simulink model "ASLIPrun2"  (R2015a)
settings: Solver=ode45  StartTime=0.0  StopTime=simtime  MaxStep=1e-3  RelTol=1e-4  AbsTol=1e-6
values from neighbouring files (symbols this model uses):
  a0 = 68*pi/180    (= 1.18682389136)    [smm_params.m]
  dt0 = -0.3325    [SLIPquad_params.m]
  dx0 = 0.4138    [SLIPquad_params.m]    (also in SLIPrun_params.m = 3; SLIPwalk_params.m = 2.5; smm_params.m = 5)
  dy0 = 0.1683    [SLIPquad_params.m]    (also in SLIPrun_params.m = -1; SLIPwalk_params.m = 0; smm_params.m = 0)
  g = 1    [SLIPquad_params.m]    (also in SLIPrun_params.m = 9.81; SLIPwalk_params.m = 9.81; smm_params.m = 9.81)
  J = 0.6    [SLIPquad_params.m]
  k = 20    [SLIPquad_params.m]    (also in SLIPrun_params.m = 23000; SLIPwalk_params.m = 10000; smm_params.m = 20000)
  L = sqrt( (u(3)-u(1))^2 + (u(4)-u(2))^2 )    [AnimSMR.m]    (also in SLIPquad_params.m = 0.5)
  l0 = 1    [SLIPquad_params.m]    (also in SLIPrun_params.m; SLIPwalk_params.m; smm_params.m)
  m = 1    [SLIPquad_params.m]    (also in SLIPrun_params.m = 70; SLIPwalk_params.m = 70; smm_params.m = 80)
  t0 = 0.056    [SLIPquad_params.m]
  x0 = []    [AnimQUAD.m]    (also in AnimQUAD2.m; AnimSMR.m; SLIPquad_params.m = 0; SLIPrun_params.m = -l*sin(theta_th))
  y0 = 1.0237    [SLIPquad_params.m]    (also in SLIPrun_params.m = sqrt(l^2 - x0^2); SLIPwalk_params.m = sqrt(l0^2 - x0^2); smm_params.m = 1)
libraries: simulink_extras x1
settings Model: Creator=hgeyer  LastModifiedBy=Joe
settings DataIOCC: SignalLoggingSaveFormat=ModelDataLogs
settings OptimizationCC: ExpressionDepthLimit=2147483647
settings DebuggingCC: UnderspecifiedInitializationDetection=Classic  MergeDetectMultiDrivingBlocksExec=none  SolverPrmCheckMsg=warning  FcnCallInpInsideContextMsg=EnableAllAsWarning  StateNameClashWarn=warning

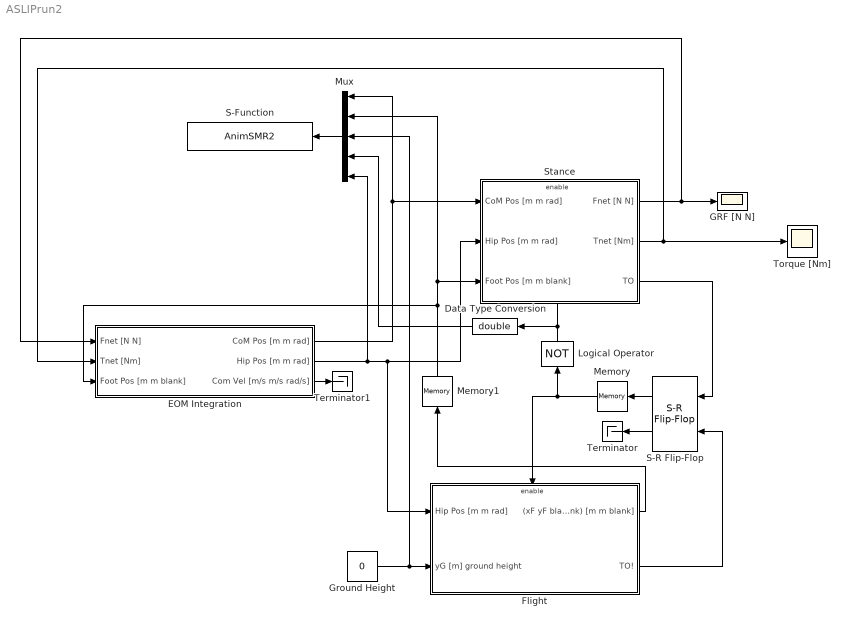
== system ASLIPrun2 ==
  Data Type Conversion : DataTypeConversion  OutDataTypeStr=double
  EOM Integration : Subsystem
  Flight : Subsystem
  GRF [N N] : Scope
      settings: YMin=-10  YMax=10
  Ground Height : Constant  Value=0
  Logical Operator : Logic  Operator=NOT  AllPortsSameDT=off  OutDataTypeStr=boolean
  Memory : Memory  X0=1
  Memory1 : Memory  X0=[0 0 0]
  Mux : Mux  Inputs=5
  S-Function : S-Function  FunctionName=AnimSMR2  Parameters=0.002
  S-R Flip-Flop : simulink_extras/Flip Flops/S-R Flip-Flop  initial_condition=1
  Stance : Subsystem
  Terminator : Terminator
  Terminator1 : Terminator
  Torque [Nm] : Scope
      settings: YMin=-10  YMax=10  SaveName=ScopeData3
  wires:
  EOM Integration/1(CoM Pos [m m rad]) -> Stance/1("CoM Pos [m m rad] "), Mux/1
  Stance/3(TO) -> S-R Flip-Flop/1
  S-R Flip-Flop/1 -> Memory/1
  Logical Operator/1 -> Data Type Conversion/1, Stance/Enable
  Memory/1 -> Logical Operator/1, Flight/Enable
  Flight/2(TO!) -> S-R Flip-Flop/2
  Stance/1(Fnet [N N]) -> EOM Integration/1(Fnet [N N]), GRF [N N]/1
  Flight/1((xF yF blank) [m m blank]) -> Memory1/1
  Memory1/1 -> EOM Integration/3(Foot Pos [m m blank]), Mux/2, Stance/3(Foot Pos [m m blank])
  Mux/1 -> S-Function/1
  S-R Flip-Flop/2 -> Terminator/1
  Ground Height/1 -> Mux/3, Flight/2(yG [m] ground height)
  EOM Integration/3(Com Vel [m/s m/s rad/s]) -> Terminator1/1
  Data Type Conversion/1 -> Mux/4
  EOM Integration/2(Hip Pos [m m rad]) -> Mux/5, Stance/2(Hip Pos [m m rad]), Flight/1(Hip Pos [m m rad])
  Stance/2(Tnet [Nm]) -> Torque [Nm]/1, EOM Integration/2(Tnet [Nm])

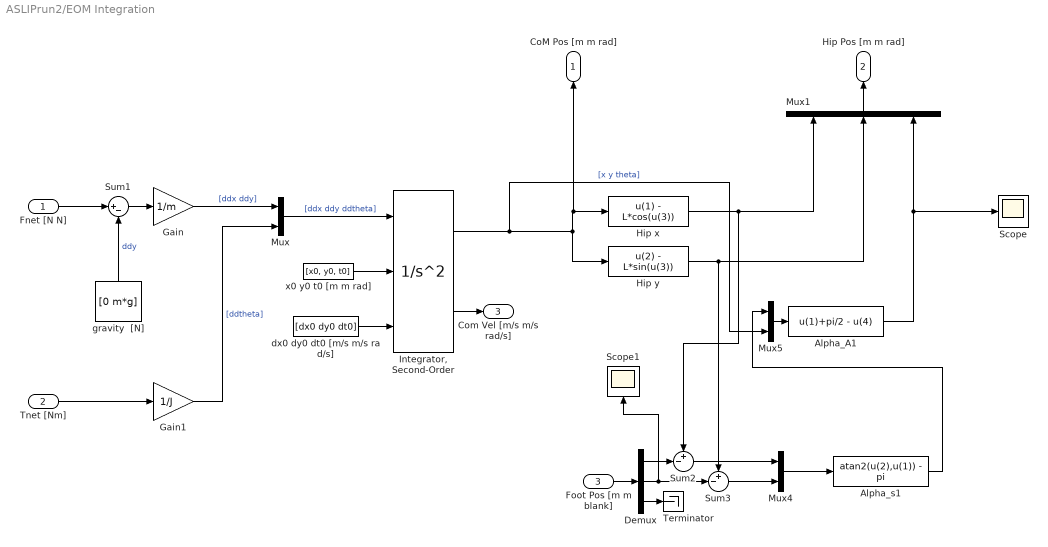
== system ASLIPrun2/EOM Integration ==
  Fnet [N N] : Inport
  Tnet [Nm] : Inport  Port=2
  Foot Pos [m m blank] : Inport  Port=3
  Alpha_A1 : Fcn  Expr=u(1)+pi/2 - u(4)
  Alpha_s1 : Fcn  Expr=atan2(u(2),u(1)) - pi
  Demux : Demux  Outputs=3
  Gain : Gain  Gain=1/m
  Gain1 : Gain  Gain=1/J
  Hip x : Fcn  Expr=u(1) - L*cos(u(3))
  Hip y : Fcn  Expr=u(2) - L*sin(u(3))
  "Integrator, Second-Order" : SecondOrderIntegrator  ICSourceX=external  ICSourceDXDT=external
  Mux : Mux  Inputs=2
  Mux1 : Mux  Inputs=3
  Mux4 : Mux  Inputs=2
  Mux5 : Mux  Inputs=2
  Scope : Scope
      settings: SaveName=ScopeData2
  Scope1 : Scope
  Sum1 : Sum  Inputs=|+-
  Sum2 : Sum  Inputs=+-|
  Sum3 : Sum  Inputs=+-|
  Terminator : Terminator
  dx0 dy0 dt0 [m/s m/s ra d/s] : Constant  Value=[dx0 dy0 dt0]
  gravity  [N] : Constant  Value=[0 m*g]
  x0 y0 t0 [m m rad] : Constant  Value=[x0, y0, t0]
  CoM Pos [m m rad] : Outport
  Hip Pos [m m rad] : Outport  Port=2
  Com Vel [m/s m/s rad/s] : Outport  Port=3
  wires:
  Sum1/1 -> Gain/1
  gravity  [N]/1 -> Sum1/2  "ddy"
  x0 y0 t0 [m m rad]/1 -> "Integrator, Second-Order"/2
  Gain/1 -> Mux/1  "[ddx ddy]"
  Fnet [N N]/1 -> Sum1/1
  dx0 dy0 dt0 [m/s m/s ra d/s]/1 -> "Integrator, Second-Order"/3
  Mux/1 -> "Integrator, Second-Order"/1  "[ddx ddy ddtheta]"
  Gain1/1 -> Mux/2  "[ddtheta]"
  Tnet [Nm]/1 -> Gain1/1
  Mux1/1 -> Hip Pos [m m rad]/1
  "Integrator, Second-Order"/2 -> Com Vel [m/s m/s rad/s]/1
  "Integrator, Second-Order"/1 -> Mux5/2, CoM Pos [m m rad]/1, Hip x/1, Hip y/1  "[x y theta]"
  Hip x/1 -> Sum2/1, Mux1/1
  Hip y/1 -> Sum3/1, Mux1/2
  Mux4/1 -> Alpha_s1/1
  Mux5/1 -> Alpha_A1/1
  Alpha_s1/1 -> Mux5/1
  Foot Pos [m m blank]/1 -> Demux/1
  Demux/2 -> Sum3/2, Scope1/1
  Demux/1 -> Sum2/2
  Sum3/1 -> Mux4/2
  Sum2/1 -> Mux4/1
  Alpha_A1/1 -> Mux1/3, Scope/1
  Demux/3 -> Terminator/1

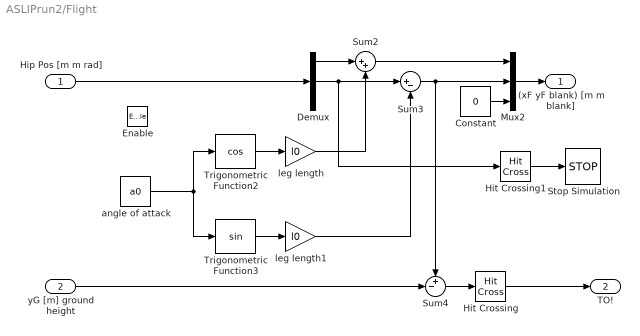
== system ASLIPrun2/Flight ==
  Hip Pos [m m rad] : Inport
  yG [m] ground height : Inport  Port=2
  Enable : EnablePort  StatesWhenEnabling=reset
  Constant : Constant  Value=0
  Demux : Demux  Outputs=3
  Hit Crossing : HitCross  HitCrossingDirection=falling
  Hit Crossing1 : HitCross  HitCrossingDirection=falling
  Mux2 : Mux  Inputs=3
  Stop Simulation : Stop
  Sum2 : Sum  Inputs=|++
  Sum3 : Sum  Inputs=|+-
  Sum4 : Sum  Inputs=+-|
  Trigonometric Function2 : Trigonometry  Operator=cos
  Trigonometric Function3 : Trigonometry
  angle of attack : Constant  Value=a0
  leg length : Gain  Gain=l0
  leg length1 : Gain  Gain=l0
  (xF yF blank) [m m blank] : Outport  InitialOutput=[0 0 0]
      settings: AttributesFormatString=%<OutputWhenDisabled>
  TO! : Outport  Port=2  OutputWhenDisabled=reset  InitialOutput=0
      settings: AttributesFormatString=%<OutputWhenDisabled>
  wires:
  Hit Crossing/1 -> TO!/1
  Demux/2 -> Hit Crossing1/1, Sum3/1
  Demux/1 -> Sum2/1
  angle of attack/1 -> Trigonometric Function3/1, Trigonometric Function2/1
  Trigonometric Function2/1 -> leg length/1
  Trigonometric Function3/1 -> leg length1/1
  Hip Pos [m m rad]/1 -> Demux/1
  leg length/1 -> Sum2/2
  leg length1/1 -> Sum3/2
  Sum3/1 -> Mux2/2, Sum4/1
  Sum2/1 -> Mux2/1
  Mux2/1 -> (xF yF blank) [m m blank]/1
  yG [m] ground height/1 -> Sum4/2
  Sum4/1 -> Hit Crossing/1
  Constant/1 -> Mux2/3
  Hit Crossing1/1 -> Stop Simulation/1

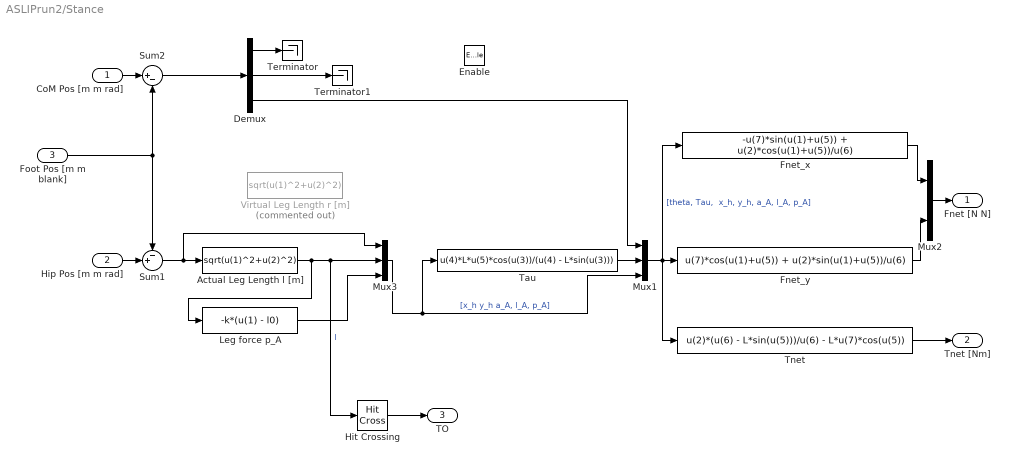
== system ASLIPrun2/Stance ==
  "CoM Pos [m m rad] " : Inport
  Hip Pos [m m rad] : Inport  Port=2
  Foot Pos [m m blank] : Inport  Port=3
  Enable : EnablePort  StatesWhenEnabling=reset
  Actual Leg Length l [m] : Fcn  Expr=sqrt(u(1)^2+u(2)^2)
  Demux : Demux  Outputs=3
  Fnet_x : Fcn  Expr=-u(7)*sin(u(1)+u(5)) + u(2)*cos(u(1)+u(5))/u(6)
  Fnet_y : Fcn  Expr=u(7)*cos(u(1)+u(5)) + u(2)*sin(u(1)+u(5))/u(6)
  Hit Crossing : HitCross  HitCrossingOffset=l0  HitCrossingDirection=rising
  Leg force p_A : Fcn  Expr=-k*(u(1) - l0)
  Mux1 : Mux  Inputs=3
  Mux2 : Mux  Inputs=2
  Mux3 : Mux  Inputs=3
  Sum1 : Sum  Inputs=-+|
  Sum2 : Sum  Inputs=|+-
  Tau : Fcn  Expr=u(4)*L*u(5)*cos(u(3))/(u(4) - L*sin(u(3)))
  Terminator : Terminator
  Terminator1 : Terminator
  Tnet : Fcn  Expr=u(2)*(u(6) - L*sin(u(5)))/u(6) - L*u(7)*cos(u(5))
  Virtual Leg Length r [m] : Fcn  Commented=on  Expr=sqrt(u(1)^2+u(2)^2)
  Fnet [N N] : Outport  OutputWhenDisabled=reset  InitialOutput=[0,0]
  Tnet [Nm] : Outport  Port=2  OutputWhenDisabled=reset  InitialOutput=[0]
  TO : Outport  Port=3  OutputWhenDisabled=reset  InitialOutput=[0]
  wires:
  Leg force p_A/1 -> Mux3/3
  Mux3/1 -> Mux1/3, Tau/1  "[x_h y_h a_A, l_A, p_A]"
  Tau/1 -> Mux1/2
  Demux/3 -> Mux1/1
  Fnet_y/1 -> Mux2/2
  Fnet_x/1 -> Mux2/1
  Mux2/1 -> Fnet [N N]/1
  Tnet/1 -> Tnet [Nm]/1
  Actual Leg Length l [m]/1 -> Hit Crossing/1, Mux3/2, Leg force p_A/1  "l"
  Hit Crossing/1 -> TO/1
  Sum2/1 -> Demux/1
  "CoM Pos [m m rad] "/1 -> Sum2/1
  Sum1/1 -> Mux3/1, Actual Leg Length l [m]/1
  Hip Pos [m m rad]/1 -> Sum1/2
  Mux1/1 -> Tnet/1, Fnet_x/1, Fnet_y/1  "[theta, Tau,  x_h, y_h, a_A, l_A, p_A]"
  Foot Pos [m m blank]/1 -> Sum2/2, Sum1/1
  Demux/1 -> Terminator/1
  Demux/2 -> Terminator1/1
